simulink model "modelX2"  (R2020b)
settings: Solver=VariableStepAuto  StartTime=0.0  StopTime=140  RelTol=1e-3
undefined symbols (not defined in the file or in its folder): f0, J, lm, psi_1, psi_2
settings Model: Creator=Acer  LastModifiedBy=Acer

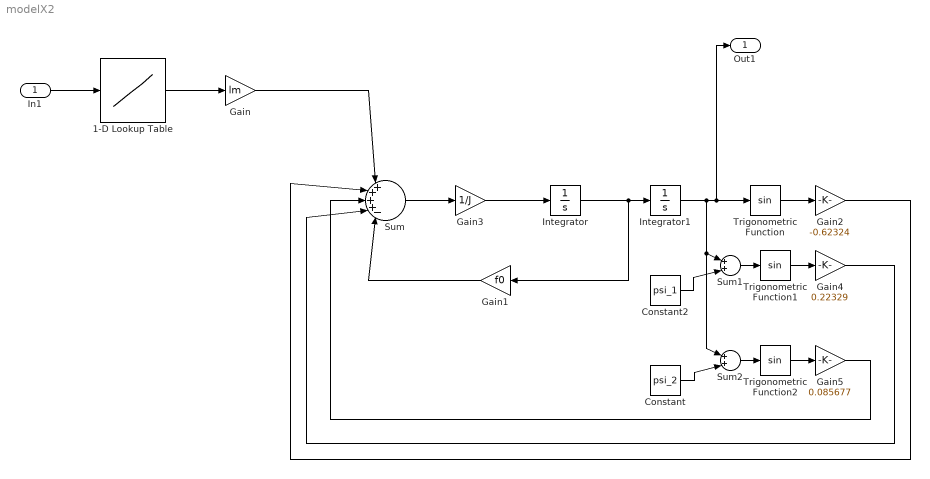
== system modelX2 ==
  In1 : Inport
  1-D Lookup Table : Lookup_n-D  NumberOfTableDimensions=1  BreakpointsForDimension1=[0,4.6, 4.7, 5, 5.5, 6, 7, 7.5, 8, 8.5, 10]  Table=[0,0,0.10984,0.21163,0.38639,0.54977,0.83,0.9284,0.9284, 0.9284,0.9284]  InternalRulePriority=Speed  RndMeth=Simplest  InputSameDT=on
  Constant : Constant  Value=psi_2
  Constant2 : Constant  Value=psi_1
  Gain : Gain  Gain=lm
  Gain1 : Gain  Gain=f0
  Gain2 : Gain  Gain=-0.62324
  Gain3 : Gain  Gain=1/J
  Gain4 : Gain  Gain=0.22329
  Gain5 : Gain  Gain=0.085677
  Integrator : Integrator
  Integrator1 : Integrator
  Sum : Sum  Inputs=|++++-|
  Sum1 : Sum  Inputs=|++|
  Sum2 : Sum  Inputs=|++|
  Trigonometric Function : Trigonometry
  Trigonometric Function1 : Trigonometry
  Trigonometric Function2 : Trigonometry
  Out1 : Outport
  wires:
  1-D Lookup Table/1 -> Gain/1
  Integrator/1 -> Integrator1/1, Gain1/1
  Sum2/1 -> Trigonometric Function2/1
  Constant2/1 -> Sum1/2
  Sum/1 -> Gain3/1
  Trigonometric Function1/1 -> Gain4/1
  Trigonometric Function/1 -> Gain2/1
  Gain5/1 -> Sum/3
  Gain4/1 -> Sum/4
  Constant/1 -> Sum2/2
  Gain3/1 -> Integrator/1
  Gain/1 -> Sum/1
  Sum1/1 -> Trigonometric Function1/1
  Gain2/1 -> Sum/2
  Trigonometric Function2/1 -> Gain5/1
  Gain1/1 -> Sum/5
  In1/1 -> 1-D Lookup Table/1
  Integrator1/1 -> Out1/1, Trigonometric Function/1, Sum2/1, Sum1/1
